simulink model "ES101A_DiagcMgr"  (R2013b)
settings: Solver=ode45  StartTime=0.0  StopTime=0.44  RelTol=1e-3
values from neighbouring files (symbols this model uses):
  BrdgVltg = DataDict.IpSignal    [ES101A_DiagcMgr_DataDict.m]
  DEM_CLEAR_PENDING = DataDict.Constant    [ES101A_DiagcMgr_DataDict.m]
  DEM_DTC_GROUP_ALL_DTCS = DataDict.Constant    [ES101A_DiagcMgr_DataDict.m]
  DFTAGICNTR_CNT_U08 = DataDict.Constant    [ES101A_DiagcMgr_DataDict.m]
  DIAGCMGR_NTCINFOSTSTESTFAILD_CNT_U08 = DataDict.Constant    [ES101A_DiagcMgrProxyX_DataDict.m]    (also in ES101A_DiagcMgr_DataDict.m)
  DIAGCMGR_NTCINFOSTSTESTFAILDTHISIGNCYC_CNT_U08 = DataDict.Constant    [ES101A_DiagcMgr_DataDict.m]
  DIAGCMGR_NTCINFOSTSTESTNOTCMPLTHISIGNCYC_CNT_U08 = DataDict.Constant    [ES101A_DiagcMgrProxyX_DataDict.m]    (also in ES101A_DiagcMgr_DataDict.m)
  DiagcMgrFltResp = DataDict.Calibration    [ES101A_DiagcMgrProxyX_DataDict.m]    (also in ES101A_DiagcMgr_DataDict.m)
  DiagcMgrNtcFltAry = DataDict.NVM    [ES101A_DiagcMgr_DataDict.m]
  DIAGCSTSCTRLDSHTDWNFLTPRSNT_CNT_U16 = DataDict.Constant    [ES101A_DiagcMgr_DataDict.m]
  DIAGCSTSDFTHWAG_CNT_U16 = DataDict.Constant    [ES101A_DiagcMgr_DataDict.m]
  DIAGCSTSDFTHWAGSERLCOMEXPRTVAL_CNT_U16 = DataDict.Constant    [ES101A_DiagcMgr_DataDict.m]
  DIAGCSTSDFTVEHSPD_CNT_U16 = DataDict.Constant    [ES101A_DiagcMgr_DataDict.m]
  DIAGCSTSININVAL_CNT_U16 = DataDict.Constant    [ES101A_DiagcMgrProxyX_DataDict.m]    (also in ES101A_DiagcMgr_DataDict.m)
  DIAGCSTSIVTR1INACTV_CNT_U16 = DataDict.Constant    [ES101A_DiagcMgr_DataDict.m]
  DIAGCSTSIVTR2INACTV_CNT_U16 = DataDict.Constant    [ES101A_DiagcMgr_DataDict.m]
  DIAGCSTSLIMDTPRFMNC_CNT_U16 = DataDict.Constant    [ES101A_DiagcMgr_DataDict.m]
  DIAGCSTSRAMPTOZEROFLTPRSNT_CNT_U16 = DataDict.Constant    [ES101A_DiagcMgr_DataDict.m]
  DIAGCSTSWHLIMBREJCTNDI_CNT_U16 = DataDict.Constant    [ES101A_DiagcMgr_DataDict.m]
  DTCIDXSTSFAIL_CNT_U08 = DataDict.Constant    [ES101A_DiagcMgr_DataDict.m]
  DTCIDXSTSNONTC_CNT_U08 = DataDict.Constant    [ES101A_DiagcMgr_DataDict.m]
  DTCIDXSTSNORES_CNT_U08 = DataDict.Constant    [ES101A_DiagcMgr_DataDict.m]
  DTCIDXSTSPASS_CNT_U08 = DataDict.Constant    [ES101A_DiagcMgr_DataDict.m]
  DTCIDXSTSUPDCFMD_CNT_U08 = DataDict.Constant    [ES101A_DiagcMgr_DataDict.m]
  ELECGLBPRM_IVTRCNT_CNT_U08 = DataDict.ConfigParam    [ES101A_DiagcMgrProxyX_DataDict.m]    (also in ES101A_DiagcMgr_DataDict.m)
  FLTINJ_DIAGCMGR_DIAGCSTSIVTR1INACTV = DataDict.Constant    [ES101A_DiagcMgr_DataDict.m]
  FLTINJ_DIAGCMGR_DIAGCSTSIVTR2INACTV = DataDict.Constant    [ES101A_DiagcMgr_DataDict.m]
  HwTq = DataDict.IpSignal    [ES101A_DiagcMgr_DataDict.m]
  IgnCntr = DataDict.IpSignal    [ES101A_DiagcMgr_DataDict.m]
  MAXDEBCNTRVAL_CNT_S16 = DataDict.Constant    [ES101A_DiagcMgr_DataDict.m]
  MAXRAMPRATE_ULSPERSEC_F32 = DataDict.Constant    [ES101A_DiagcMgrProxyX_DataDict.m]    (also in ES101A_DiagcMgr_DataDict.m)
  MINDEBCNTRVAL_CNT_S16 = DataDict.Constant    [ES101A_DiagcMgr_DataDict.m]
  MINRAMPRATE_ULSPERSEC_F32 = DataDict.Constant    [ES101A_DiagcMgrProxyX_DataDict.m]    (also in ES101A_DiagcMgr_DataDict.m)
  SCAMOTTQCMDTOONE_ULS_F32 = DataDict.Constant    [ES101A_DiagcMgrProxyX_DataDict.m]    (also in ES101A_DiagcMgr_DataDict.m)
  SCAMOTTQCMDTOZERO_ULS_F32 = DataDict.Constant    [ES101A_DiagcMgrProxyX_DataDict.m]    (also in ES101A_DiagcMgr_DataDict.m)
  SysSt = DataDict.IpSignal    [ES101A_DiagcMgr_DataDict.m]
  VehSpd = DataDict.IpSignal    [ES101A_DiagcMgr_DataDict.m]
undefined symbols (not defined in the file or in its folder): ActvMotTqCmdSca, ActvRampRate, AgiCntr, Dem_DTCFormatType, Dem_DTCOriginType, Dem_EventStatusType, DiagcData, DiagcMgrNtcMap, DiagcSts, DtcEnaMask, EcuT, HistNtcFltAry, MicroDiagcData, MotTq, NtcNr, NtcNrWithResd1, NtcStInfo, ProxySetNtcData, Sts, SysSt1, TOTNROFDTC_CNT_U08
libraries: simulink x149, FloatToFixd x5, NxtrNvM x3
(part 9 of 13)

== system ES101A_DiagcMgr/DiagcMgr/SetNtcStsCore/NtcNr is Valid/Diagnostics Not Inhibited/NtcEnabled/NTCSTS_PREPASSD/Update NtcInfoSts/Do Nothing ==
  Action Port : ActionPort  ActionType=else
  CopyRight2 : Subsystem  Description=|  mask(Copyright Information){none=on}
      | Copyright info block.                                               
      |                                                                     
      | Place copyright information at the top of every subsystem in design.
      mask prompts: none "No parameters"
      mask help: Place copyright information at the top of every subsystem in design.
      mask Display:
      | NxtrConf = 'Nexteer Confidential';
      | 
      | sys = bdroot; %handle for the current model ("system")
      | first = get_param(sys,'Created');
      | first = first(end-3:end);  %year is last four digits
      | 
      | last = get_param(sys,'LastModifiedDate');
      | if isempty(last)
      |     last = datestr(now,'yyyy');
      | else
      |     last = last(end-3:end);
      | end
      | 
      | if strcmp(first,last)
      |     fprintf('%s -- Copyright %s Nexteer',NxtrConf,first)
      | else
      |     fprintf('%s -- %s%s- %s Nexteer',NxtrConf,char(169),first,last)
      | end

== system ES101A_DiagcMgr/DiagcMgr/SetNtcStsCore/NtcNr is Valid/Diagnostics Not Inhibited/NtcEnabled/NTCSTS_PREPASSD/Update NtcInfoSts/Update NTC Info's Status Byte & Update the NTC Fault Array ==
  NtcInfo_ArgIn : Inport
  DebStep_ArgIn : Inport  Port=2
  NtcInfoDebCntr_ArgIn : Inport  Port=3
  Action Port : ActionPort  ActionType=then
  CopyRight2 : Subsystem  Description=|  mask(Copyright Information){none=on}
      | Copyright info block.                                               
      |                                                                     
      | Place copyright information at the top of every subsystem in design.
      mask prompts: none "No parameters"
      mask help: Place copyright information at the top of every subsystem in design.
      mask Display:
      | NxtrConf = 'Nexteer Confidential';
      | 
      | sys = bdroot; %handle for the current model ("system")
      | first = get_param(sys,'Created');
      | first = first(end-3:end);  %year is last four digits
      | 
      | last = get_param(sys,'LastModifiedDate');
      | if isempty(last)
      |     last = datestr(now,'yyyy');
      | else
      |     last = last(end-3:end);
      | end
      | 
      | if strcmp(first,last)
      |     fprintf('%s -- Copyright %s Nexteer',NxtrConf,first)
      | else
      |     fprintf('%s -- %s%s- %s Nexteer',NxtrConf,char(169),first,last)
      | end
  Decrement Counter : Subsystem  RequirementInfo="{'linktype_rmi_doors' '0000c474 (/ESG Group/FDD Module Requirements/EA4 Specific/ES101A_DiagcMgr)' '#ES101A_271' 'true' 'REQ:  ES101A_271' '' ; 'linktype_rmi_doors' '0000c474 (/ESG Group/FDD Module Requirements/EA4 Specific/ES101A_DiagcMgr)' '#ES101A_272' 'true' 'REQ:  ES101A_272' '' } %GIDa_7e8fb58f_d104_4b81_a44a_d0c429ffb579"  Priority=1  TreatAsAtomicUnit=on
      settings: AttributesFormatString=Priority = %<Priority>  RTWSystemCode=Inline
  "NtcInfo_ArgOut " : Outport
  NtcInfoDebCntr_ArgOut : Outport  Port=2
  wires:
  Decrement Counter/1(NtcInfo_ArgOut) -> "NtcInfo_ArgOut "/1
  DebStep_ArgIn/1 -> Decrement Counter/2(DebStep_ArgIn)
  NtcInfo_ArgIn/1 -> Decrement Counter/1("NtcInfo_ArgIn ")
  NtcInfoDebCntr_ArgIn/1 -> Decrement Counter/3(NtcInfoDebCntr_ArgIn)
  Decrement Counter/2(NtcInfoDebCntr_ArgOut) -> NtcInfoDebCntr_ArgOut/1

== system ES101A_DiagcMgr/DiagcMgr/DiagcMgrIninCore/Update NtcInfoAry From NvM/Update NtcInfoAry/Update NtcInfoAry Aging Counter And Confirmed Bit/If Action/Subsystem/0 < AgingCntr < 64/CopyRight2 ==

== system ES101A_DiagcMgr/DiagcMgr/DiagcMgrIninCore/Update NtcInfoAry From NvM/Update NtcInfoAry/Update NtcInfoAry Aging Counter And Confirmed Bit/If Action/Subsystem/AgingCntr >= 64 Do Nothing/CopyRight1 ==

== system ES101A_DiagcMgr/DiagcMgr/DiagcMgrPer2/Normal Periodic Processing/For All DTCs/For Each DTC/Check If DTC Status has Changed/DTC Status Changed OR DTC Update NOT Confirmed/Update DTC Index Previous Status with DTC Index Current Status/CopyRight2 ==

== system ES101A_DiagcMgr/DiagcMgr/DiagcMgrPer2/Normal Periodic Processing/For All DTCs/For Each DTC/Check If DTC Status has Changed/DTC Status Changed OR DTC Update NOT Confirmed/Update DTC Status/CopyRight2 ==

== system ES101A_DiagcMgr/DiagcMgr/DiagcMgrPer2/Normal Periodic Processing/For All DTCs/For Each DTC/Check If DTC Status has Changed/DTC Status Changed OR DTC Update NOT Confirmed/Update DTC Status/Dtc Status is Failed ==
  DtcIdx : Inport
  Action Port : ActionPort  ActionType=elseif
  Constant1 : Constant  Value=Dem_EventStatusType.DEM_EVENT_STATUS_FAILED
  CopyRight2 : Subsystem  Description=|  mask(Copyright Information){none=on}
      | Copyright info block.                                               
      |                                                                     
      | Place copyright information at the top of every subsystem in design.
      mask prompts: none "No parameters"
      mask help: Place copyright information at the top of every subsystem in design.
      mask Display:
      | NxtrConf = 'Nexteer Confidential';
      | 
      | sys = bdroot; %handle for the current model ("system")
      | first = get_param(sys,'Created');
      | first = first(end-3:end);  %year is last four digits
      | 
      | last = get_param(sys,'LastModifiedDate');
      | if isempty(last)
      |     last = datestr(now,'yyyy');
      | else
      |     last = last(end-3:end);
      | end
      | 
      | if strcmp(first,last)
      |     fprintf('%s -- Copyright %s Nexteer',NxtrConf,first)
      | else
      |     fprintf('%s -- %s%s- %s Nexteer',NxtrConf,char(169),first,last)
      | end
  Data Store Read : DataStoreRead  DataStoreName=DemDtcEveIdMap
  Dem_SetEventStatus : Subsystem
  Selector2 : Selector  IndexMode=Zero-based  InputPortWidth=14  IndexOptions=Index vector (port)  Indices=[1 3]  OutputSizes=1
  Update 'DTC Index Update Confirmed' Bit : Subsystem
  wires:
  Dem_SetEventStatus/1(Dem_SetEventStatus_StdRtn) -> Update 'DTC Index Update Confirmed' Bit/1(Dem_SetEventStatus_StdRtn)
  Constant1/1 -> Dem_SetEventStatus/2(EventStatus), Update 'DTC Index Update Confirmed' Bit/2(DtcIdxPrevSts)
  Data Store Read/1 -> Selector2/1
  Selector2/1 -> Dem_SetEventStatus/1(EventId)
  DtcIdx/1 -> Selector2/2, Update 'DTC Index Update Confirmed' Bit/3(DtcIdx)

== system ES101A_DiagcMgr/DiagcMgr/DiagcMgrPer2/Normal Periodic Processing/For All DTCs/For Each DTC/Check If DTC Status has Changed/DTC Status Changed OR DTC Update NOT Confirmed/Update DTC Status/Dtc Status is No Result or No Ntc ==
  DtcIdx : Inport
  Action Port : ActionPort
  Assignment : Assignment  IndexMode=Zero-based  IndexOptions=Starting index (port)  Indices=1  OutputSizes=1
  CopyRight2 : Subsystem  Description=|  mask(Copyright Information){none=on}
      | Copyright info block.                                               
      |                                                                     
      | Place copyright information at the top of every subsystem in design.
      mask prompts: none "No parameters"
      mask help: Place copyright information at the top of every subsystem in design.
      mask Display:
      | NxtrConf = 'Nexteer Confidential';
      | 
      | sys = bdroot; %handle for the current model ("system")
      | first = get_param(sys,'Created');
      | first = first(end-3:end);  %year is last four digits
      | 
      | last = get_param(sys,'LastModifiedDate');
      | if isempty(last)
      |     last = datestr(now,'yyyy');
      | else
      |     last = last(end-3:end);
      | end
      | 
      | if strcmp(first,last)
      |     fprintf('%s -- Copyright %s Nexteer',NxtrConf,first)
      | else
      |     fprintf('%s -- %s%s- %s Nexteer',NxtrConf,char(169),first,last)
      | end
  Data Store Read : DataStoreRead  DataStoreName=DtcIdxPrevSts
  Data Store Read1 : DataStoreRead  DataStoreName=DtcIdxPrevSts
  Data Store Write : DataStoreWrite  DataStoreName=DtcIdxPrevSts
  Set Bit 7 (DTC Update Confirmed) : Subsystem
  wires:
  Data Store Read/1 -> Assignment/1
  Assignment/1 -> Data Store Write/1
  DtcIdx/1 -> Assignment/3
  Data Store Read1/1 -> Set Bit 7 (DTC Update Confirmed)/1(In1)
  Set Bit 7 (DTC Update Confirmed)/1(Out1) -> Assignment/2

== system ES101A_DiagcMgr/DiagcMgr/DiagcMgrPer2/Normal Periodic Processing/For All DTCs/For Each DTC/Check If DTC Status has Changed/DTC Status Changed OR DTC Update NOT Confirmed/Update DTC Status/Dtc Status is Passed ==
  DtcIdx : Inport
  Action Port : ActionPort
  Constant : Constant  Value=Dem_EventStatusType.DEM_EVENT_STATUS_PASSED
  CopyRight2 : Subsystem  Description=|  mask(Copyright Information){none=on}
      | Copyright info block.                                               
      |                                                                     
      | Place copyright information at the top of every subsystem in design.
      mask prompts: none "No parameters"
      mask help: Place copyright information at the top of every subsystem in design.
      mask Display:
      | NxtrConf = 'Nexteer Confidential';
      | 
      | sys = bdroot; %handle for the current model ("system")
      | first = get_param(sys,'Created');
      | first = first(end-3:end);  %year is last four digits
      | 
      | last = get_param(sys,'LastModifiedDate');
      | if isempty(last)
      |     last = datestr(now,'yyyy');
      | else
      |     last = last(end-3:end);
      | end
      | 
      | if strcmp(first,last)
      |     fprintf('%s -- Copyright %s Nexteer',NxtrConf,first)
      | else
      |     fprintf('%s -- %s%s- %s Nexteer',NxtrConf,char(169),first,last)
      | end
  Data Store Read : DataStoreRead  DataStoreName=DemDtcEveIdMap
  Dem_SetEventStatus : Subsystem
  Selector2 : Selector  IndexMode=Zero-based  InputPortWidth=14  IndexOptions=Index vector (port)  Indices=[1 3]  OutputSizes=1
  Update 'DTC Index Update Confirmed' Bit : Subsystem
  wires:
  Constant/1 -> Update 'DTC Index Update Confirmed' Bit/2(DtcIdxPrevSts), Dem_SetEventStatus/2(EventStatus)
  Dem_SetEventStatus/1(Dem_SetEventStatus_StdRtn) -> Update 'DTC Index Update Confirmed' Bit/1(Dem_SetEventStatus_StdRtn)
  DtcIdx/1 -> Update 'DTC Index Update Confirmed' Bit/3(DtcIdx), Selector2/2
  Selector2/1 -> Dem_SetEventStatus/1(EventId)
  Data Store Read/1 -> Selector2/1

== system ES101A_DiagcMgr/DiagcMgr/DiagcMgrPer2/Normal Periodic Processing/For All NTCs/For Each NTC/Update DTC Status/NTC Enabled/DTC Fail/CopyRight2 ==

== system ES101A_DiagcMgr/DiagcMgr/DiagcMgrPer2/Normal Periodic Processing/For All NTCs/For Each NTC/Update DTC Status/NTC Enabled/DTC NoRes/CopyRight2 ==

== system ES101A_DiagcMgr/DiagcMgr/DiagcMgrPer2/Normal Periodic Processing/For All NTCs/For Each NTC/Update DTC Status/NTC Enabled/DTC Pass/CopyRight2 ==

== system ES101A_DiagcMgr/DiagcMgr/DiagcMgrPer2/Normal Periodic Processing/For All NTCs/For Each NTC/Update DTC Status/NTC Enabled/Do Nothing/CopyRight2 ==

== system ES101A_DiagcMgr/DiagcMgr/SetNtcStsCore/NtcNr is Valid/Diagnostics Not Inhibited/NtcEnabled/NTCSTS_FAILD/Update ISO Bits, Parameter Byte and AgiCntr /ProcessRampResponse and DiagcSts/ControlledShutdown Fault ==
  DiagcData_ArgIn : Inport
  ProxySetNtcData_ArgIn : Inport  Port=2
  TmpDiagcSts : Inport  Port=3
  Action Port : ActionPort
  Atomic Section2 : Subsystem  Description=|  RequirementInfo="{'linktype_rmi_doors' '0000c474 (/ESG Group/FDD Module Requirements/EA4 Specific/ES101A_DiagcMgr)' '#ES101A_300' 'true' 'REQ:  ES101A_300' '' } %GIDa_2bc6450b_700c_4982_9445_5c86aef287c5"
      | EXCLUSIVE AREA:
      | Write data into the DiagcSts Register & ActvRampRate Register
      settings: AttributesFormatString=%<Description>
  Bitwise Operator : simulink/Logic and Bit Operations/Bitwise Operator  logicop=OR  UseBitMask=off  NumInputPorts=3  BitMask=bin2dec('11011001')  BitMaskRealWorld=Stored Integer
  CopyRight2 : Subsystem  Description=|  mask(Copyright Information){none=on}
      | Copyright info block.                                               
      |                                                                     
      | Place copyright information at the top of every subsystem in design.
      mask prompts: none "No parameters"
      mask help: Place copyright information at the top of every subsystem in design.
      mask Display:
      | NxtrConf = 'Nexteer Confidential';
      | 
      | sys = bdroot; %handle for the current model ("system")
      | first = get_param(sys,'Created');
      | first = first(end-3:end);  %year is last four digits
      | 
      | last = get_param(sys,'LastModifiedDate');
      | if isempty(last)
      |     last = datestr(now,'yyyy');
      | else
      |     last = last(end-3:end);
      | end
      | 
      | if strcmp(first,last)
      |     fprintf('%s -- Copyright %s Nexteer',NxtrConf,first)
      | else
      |     fprintf('%s -- %s%s- %s Nexteer',NxtrConf,char(169),first,last)
      | end
  Diagnostic Status Controlled Shutdown Fault Present : Constant  Value=DIAGCSTSCTRLDSHTDWNFLTPRSNT_CNT_U16
  Ramp To Zero Fault Present : Constant  Value=DIAGCSTSRAMPTOZEROFLTPRSNT_CNT_U16  OutDataTypeStr=uint16
  DiagcData_ArgOut : Outport
  ProxySetNtcData_ArgOut : Outport  Port=2
  wires:
  Diagnostic Status Controlled Shutdown Fault Present/1 -> Bitwise Operator/1
  Ramp To Zero Fault Present/1 -> Bitwise Operator/2
  Bitwise Operator/1 -> Atomic Section2/1(TmpDiagcSts)
  DiagcData_ArgIn/1 -> Atomic Section2/2(DiagcData_ArgInOut)
  ProxySetNtcData_ArgIn/1 -> Atomic Section2/3(ProxySetNtcData_ArgInOut)
  Atomic Section2/1(DiagcData_ArgOut) -> DiagcData_ArgOut/1
  Atomic Section2/2(ProxySetNtcData_ArgOut) -> ProxySetNtcData_ArgOut/1
  TmpDiagcSts/1 -> Bitwise Operator/3

== system ES101A_DiagcMgr/DiagcMgr/SetNtcStsCore/NtcNr is Valid/Diagnostics Not Inhibited/NtcEnabled/NTCSTS_FAILD/Update ISO Bits, Parameter Byte and AgiCntr /ProcessRampResponse and DiagcSts/CopyRight2 ==

== system ES101A_DiagcMgr/DiagcMgr/SetNtcStsCore/NtcNr is Valid/Diagnostics Not Inhibited/NtcEnabled/NTCSTS_FAILD/Update ISO Bits, Parameter Byte and AgiCntr /ProcessRampResponse and DiagcSts/InformationOnly Fault ==
  DiagcData_ArgIn : Inport
  ProxySetNtcData_ArgIn : Inport  Port=2
  TmpDiagcSts : Inport  Port=3
  Action Port : ActionPort
  Atomic Section2 : Subsystem  Description=|  RequirementInfo="{'linktype_rmi_doors' '0000c474 (/ESG Group/FDD Module Requirements/EA4 Specific/ES101A_DiagcMgr)' '#ES101A_300' 'true' 'REQ:  ES101A_300' '' } %GIDa_9448650f_4c83_4875_bae7_9fccd1156efd"
      | EXCLUSIVE AREA:
      | Write data into the DiagcSts Register & ActvRampRate Register
      settings: AttributesFormatString=%<Description>
  CopyRight2 : Subsystem  Description=|  mask(Copyright Information){none=on}
      | Copyright info block.                                               
      |                                                                     
      | Place copyright information at the top of every subsystem in design.
      mask prompts: none "No parameters"
      mask help: Place copyright information at the top of every subsystem in design.
      mask Display:
      | NxtrConf = 'Nexteer Confidential';
      | 
      | sys = bdroot; %handle for the current model ("system")
      | first = get_param(sys,'Created');
      | first = first(end-3:end);  %year is last four digits
      | 
      | last = get_param(sys,'LastModifiedDate');
      | if isempty(last)
      |     last = datestr(now,'yyyy');
      | else
      |     last = last(end-3:end);
      | end
      | 
      | if strcmp(first,last)
      |     fprintf('%s -- Copyright %s Nexteer',NxtrConf,first)
      | else
      |     fprintf('%s -- %s%s- %s Nexteer',NxtrConf,char(169),first,last)
      | end
  DiagcData_ArgOut : Outport
  ProxySetNtcData_ArgOut : Outport  Port=2
  wires:
  DiagcData_ArgIn/1 -> Atomic Section2/1(DiagcData_ArgInOut)
  ProxySetNtcData_ArgIn/1 -> Atomic Section2/2(ProxySetNtcData_ArgInOut)
  Atomic Section2/1(DiagcData_ArgOut) -> DiagcData_ArgOut/1
  Atomic Section2/2(ProxySetNtcData_ArgOut) -> ProxySetNtcData_ArgOut/1
  TmpDiagcSts/1 -> Atomic Section2/3(TmpDiagcSts)

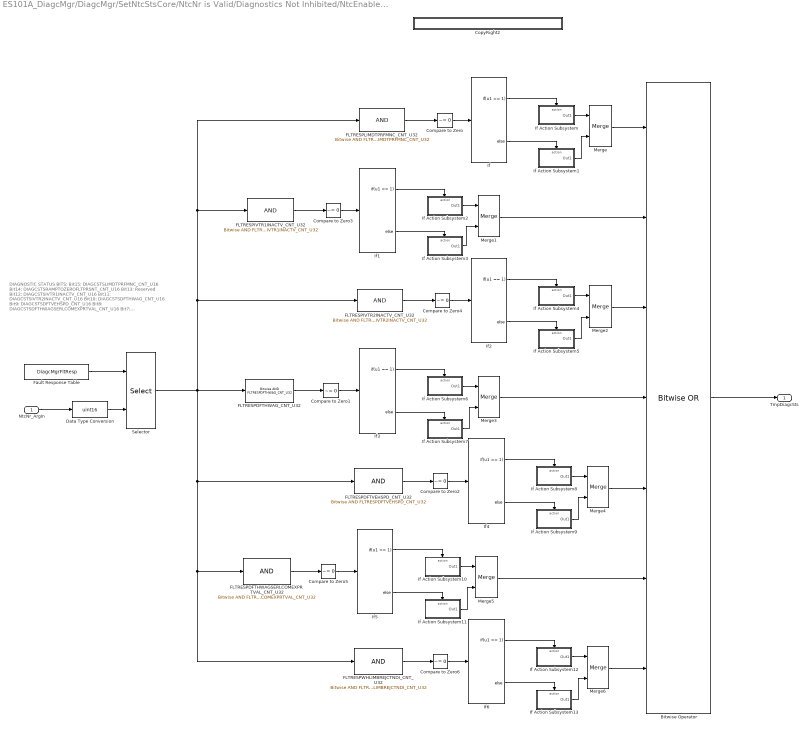
== system ES101A_DiagcMgr/DiagcMgr/SetNtcStsCore/NtcNr is Valid/Diagnostics Not Inhibited/NtcEnabled/NTCSTS_FAILD/Update ISO Bits, Parameter Byte and AgiCntr /ProcessRampResponse and DiagcSts/ProcessDiagcSts ==
  note: DIAGNOSTIC  STATUS  BITS:
      |
      | Bit15: DIAGCSTSLIMDTPRFMNC_CNT_U16
      | Bit14: DIAGCSTSRAMPTOZEROFLTPRSNT_CNT_U16
      | Bit13: Reserved
      | Bit12: DIAGCSTSIVTR1INACTV_CNT_U16
      | Bit11: DIAGCSTSIVTR2INACTV_CNT_U16
      | Bit10: DIAGCSTSDFTHWAG_CNT_U16
      | Bit9:   DIAGCSTSDFTVEHSPD_CNT_U16
      | Bit8:   DIAGCSTSDFTHWAGSERLCOMEXPRTVAL_CNT_U16
      | Bit7:   DIAGCSTSWHLIMBREJCTNDI_CNT_U16
      | Bit6:	   DIAGCSTSCTRLDIRAMP_CNT_U16
  NtcNr_ArgIn : Inport
  Bitwise Operator : simulink/Logic and Bit Operations/Bitwise Operator  logicop=OR  UseBitMask=off  NumInputPorts=7  BitMask=bin2dec('11011001')  BitMaskRealWorld=Stored Integer
  Compare to Zero{,1..6} (7 alike) : simulink/Logic and Bit Operations/Compare To Zero  relop=~=  OutDataTypeStr=boolean
  CopyRight2 : Subsystem  Description=|  mask(Copyright Information){none=on}
      | Copyright info block.                                               
      |                                                                     
      | Place copyright information at the top of every subsystem in design.
      mask prompts: none "No parameters"
      mask help: Place copyright information at the top of every subsystem in design.
      mask Display:
      | NxtrConf = 'Nexteer Confidential';
      | 
      | sys = bdroot; %handle for the current model ("system")
      | first = get_param(sys,'Created');
      | first = first(end-3:end);  %year is last four digits
      | 
      | last = get_param(sys,'LastModifiedDate');
      | if isempty(last)
      |     last = datestr(now,'yyyy');
      | else
      |     last = last(end-3:end);
      | end
      | 
      | if strcmp(first,last)
      |     fprintf('%s -- Copyright %s Nexteer',NxtrConf,first)
      | else
      |     fprintf('%s -- %s%s- %s Nexteer',NxtrConf,char(169),first,last)
      | end
  Data Type Conversion : DataTypeConversion  OutDataTypeStr=uint16
  FLTRESPDFTHWAGSERLCOMEXPRTVAL_CNT_U32 : simulink/Logic and Bit Operations/Bitwise Operator  logicop=AND  UseBitMask=on  BitMask=FLTRESPDFTHWAGSERLCOMEXPRTVAL_CNT_U32  BitMaskRealWorld=Stored Integer
  FLTRESPDFTHWAG_CNT_U32 : simulink/Logic and Bit Operations/Bitwise Operator  logicop=AND  UseBitMask=on  BitMask=FLTRESPDFTHWAG_CNT_U32  BitMaskRealWorld=Stored Integer
  FLTRESPDFTVEHSPD_CNT_U32 : simulink/Logic and Bit Operations/Bitwise Operator  logicop=AND  UseBitMask=on  BitMask=FLTRESPDFTVEHSPD_CNT_U32  BitMaskRealWorld=Stored Integer
  FLTRESPIVTR1INACTV_CNT_U32 : simulink/Logic and Bit Operations/Bitwise Operator  RequirementInfo={} %GIDa_da088e71_cf55_4258_9e23_348948e7cf64  logicop=AND  UseBitMask=on  BitMask=FLTRESPIVTR1INACTV_CNT_U32  BitMaskRealWorld=Stored Integer
  FLTRESPIVTR2INACTV_CNT_U32 : simulink/Logic and Bit Operations/Bitwise Operator  RequirementInfo={} %GIDa_49040b40_7700_4617_a7b3_5f9f919de844  logicop=AND  UseBitMask=on  BitMask=FLTRESPIVTR2INACTV_CNT_U32  BitMaskRealWorld=Stored Integer
  FLTRESPLIMDTPRFMNC_CNT_U32 : simulink/Logic and Bit Operations/Bitwise Operator  RequirementInfo={} %GIDa_3a19e481_3aa4_478f_99c0_cab30f84ef14  logicop=AND  UseBitMask=on  BitMask=FLTRESPLIMDTPRFMNC_CNT_U32  BitMaskRealWorld=Stored Integer
  FLTRESPWHLIMBREJCTNDI_CNT_U32 : simulink/Logic and Bit Operations/Bitwise Operator  logicop=AND  UseBitMask=on  BitMask=FLTRESPWHLIMBREJCTNDI_CNT_U32  BitMaskRealWorld=Stored Integer
  Fault Response Table : Constant  Value=DiagcMgrFltResp
  If{,1..6} (7 alike) : If  IfExpression=u1 == 1
  If Action Subsystem : Subsystem  TreatAsAtomicUnit=on
  If Action Subsystem1 : Subsystem  TreatAsAtomicUnit=on
  If Action Subsystem10 : Subsystem  TreatAsAtomicUnit=on
  If Action Subsystem11 : Subsystem  TreatAsAtomicUnit=on
  If Action Subsystem12 : Subsystem  TreatAsAtomicUnit=on
  If Action Subsystem13 : Subsystem  TreatAsAtomicUnit=on
  If Action Subsystem2 : Subsystem  TreatAsAtomicUnit=on
  If Action Subsystem3 : Subsystem  TreatAsAtomicUnit=on
  If Action Subsystem4 : Subsystem  TreatAsAtomicUnit=on
  If Action Subsystem5 : Subsystem  TreatAsAtomicUnit=on
  If Action Subsystem6 : Subsystem  TreatAsAtomicUnit=on
  If Action Subsystem7 : Subsystem  TreatAsAtomicUnit=on
  If Action Subsystem8 : Subsystem  TreatAsAtomicUnit=on
  If Action Subsystem9 : Subsystem  TreatAsAtomicUnit=on
  Merge{,1..6} (7 alike) : Merge
  Selector : Selector  IndexMode=Zero-based  InputPortWidth=512  IndexOptions=Index vector (port)  Indices=[1 3]  OutputSizes=1
  TmpDiagcSts : Outport
  wires:
  Compare to Zero4/1 -> If2/1
  Merge2/1 -> Bitwise Operator/3
  If Action Subsystem5/1(Out1) -> Merge2/2
  If Action Subsystem4/1(Out1) -> Merge2/1
  If2/2 -> If Action Subsystem5/Action
  If2/1 -> If Action Subsystem4/Action
  Merge1/1 -> Bitwise Operator/2
  Compare to Zero3/1 -> If1/1
  If Action Subsystem3/1(Out1) -> Merge1/2
  If Action Subsystem2/1(Out1) -> Merge1/1
  If1/2 -> If Action Subsystem3/Action
  If1/1 -> If Action Subsystem2/Action
  Merge/1 -> Bitwise Operator/1
  If Action Subsystem1/1(Out1) -> Merge/2
  If Action Subsystem/1(Out1) -> Merge/1
  Compare to Zero/1 -> If/1
  If/2 -> If Action Subsystem1/Action
  If/1 -> If Action Subsystem/Action
  Bitwise Operator/1 -> TmpDiagcSts/1
  FLTRESPIVTR2INACTV_CNT_U32/1 -> Compare to Zero4/1
  FLTRESPIVTR1INACTV_CNT_U32/1 -> Compare to Zero3/1
  Selector/1 -> FLTRESPWHLIMBREJCTNDI_CNT_U32/1, FLTRESPDFTHWAGSERLCOMEXPRTVAL_CNT_U32/1, FLTRESPDFTVEHSPD_CNT_U32/1, FLTRESPDFTHWAG_CNT_U32/1, FLTRESPLIMDTPRFMNC_CNT_U32/1, FLTRESPIVTR1INACTV_CNT_U32/1, FLTRESPIVTR2INACTV_CNT_U32/1
  Fault Response Table/1 -> Selector/1
  NtcNr_ArgIn/1 -> Data Type Conversion/1
  FLTRESPLIMDTPRFMNC_CNT_U32/1 -> Compare to Zero/1
  Compare to Zero1/1 -> If3/1
  Merge3/1 -> Bitwise Operator/4
  If Action Subsystem7/1(Out1) -> Merge3/2
  If Action Subsystem6/1(Out1) -> Merge3/1
  If3/2 -> If Action Subsystem7/Action
  If3/1 -> If Action Subsystem6/Action
  FLTRESPDFTHWAG_CNT_U32/1 -> Compare to Zero1/1
  Compare to Zero2/1 -> If4/1
  Merge4/1 -> Bitwise Operator/5
  If Action Subsystem9/1(Out1) -> Merge4/2
  If Action Subsystem8/1(Out1) -> Merge4/1
  If4/2 -> If Action Subsystem9/Action
  If4/1 -> If Action Subsystem8/Action
  FLTRESPDFTVEHSPD_CNT_U32/1 -> Compare to Zero2/1
  Compare to Zero5/1 -> If5/1
  Merge5/1 -> Bitwise Operator/6
  If Action Subsystem11/1(Out1) -> Merge5/2
  If Action Subsystem10/1(Out1) -> Merge5/1
  If5/2 -> If Action Subsystem11/Action
  If5/1 -> If Action Subsystem10/Action
  FLTRESPDFTHWAGSERLCOMEXPRTVAL_CNT_U32/1 -> Compare to Zero5/1
  Compare to Zero6/1 -> If6/1
  Merge6/1 -> Bitwise Operator/7
  If Action Subsystem13/1(Out1) -> Merge6/2
  If Action Subsystem12/1(Out1) -> Merge6/1
  If6/2 -> If Action Subsystem13/Action
  If6/1 -> If Action Subsystem12/Action
  FLTRESPWHLIMBREJCTNDI_CNT_U32/1 -> Compare to Zero6/1
  Data Type Conversion/1 -> Selector/2

== system ES101A_DiagcMgr/DiagcMgr/SetNtcStsCore/NtcNr is Valid/Diagnostics Not Inhibited/NtcEnabled/NTCSTS_FAILD/Update ISO Bits, Parameter Byte and AgiCntr /ProcessRampResponse and DiagcSts/RapidShutdown Fault ==
  DiagcData_ArgIn : Inport
  ProxySetNtcData_ArgIn : Inport  Port=2
  TmpDiagcSts : Inport  Port=3
  Action Port : ActionPort
  Atomic Section2 : Subsystem  Description=|  RequirementInfo="{'linktype_rmi_doors' '0000c474 (/ESG Group/FDD Module Requirements/EA4 Specific/ES101A_DiagcMgr)' '#ES101A_300' 'true' 'REQ:  ES101A_300' '' } %GIDa_00cb0b6f_e255_4c4e_bed6_f3cda34ac4d2"
      | EXCLUSIVE AREA:
      | Write data into the DiagcSts Register & ActvRampRate Register
      settings: AttributesFormatString=%<Description>
  Bitwise Operator : simulink/Logic and Bit Operations/Bitwise Operator  logicop=OR  UseBitMask=off  NumInputPorts=2  BitMask=bin2dec('11011001')  BitMaskRealWorld=Stored Integer
  CopyRight2 : Subsystem  Description=|  mask(Copyright Information){none=on}
      | Copyright info block.                                               
      |                                                                     
      | Place copyright information at the top of every subsystem in design.
      mask prompts: none "No parameters"
      mask help: Place copyright information at the top of every subsystem in design.
      mask Display:
      | NxtrConf = 'Nexteer Confidential';
      | 
      | sys = bdroot; %handle for the current model ("system")
      | first = get_param(sys,'Created');
      | first = first(end-3:end);  %year is last four digits
      | 
      | last = get_param(sys,'LastModifiedDate');
      | if isempty(last)
      |     last = datestr(now,'yyyy');
      | else
      |     last = last(end-3:end);
      | end
      | 
      | if strcmp(first,last)
      |     fprintf('%s -- Copyright %s Nexteer',NxtrConf,first)
      | else
      |     fprintf('%s -- %s%s- %s Nexteer',NxtrConf,char(169),first,last)
      | end
  Ramp To Zero Fault Present1 : Constant  Value=DIAGCSTSRAMPTOZEROFLTPRSNT_CNT_U16  OutDataTypeStr=uint16
  "DiagcData_ArgOut " : Outport
  "ProxySetNtcData_ArgOut " : Outport  Port=2
  wires:
  Ramp To Zero Fault Present1/1 -> Bitwise Operator/1
  Bitwise Operator/1 -> Atomic Section2/1(TmpDiagcSts)
  TmpDiagcSts/1 -> Bitwise Operator/2
  DiagcData_ArgIn/1 -> Atomic Section2/2(DiagcData_ArgIn)
  ProxySetNtcData_ArgIn/1 -> Atomic Section2/3(ProxySetNtcData_ArgIn)
  Atomic Section2/1("DiagcData_ArgInOut ") -> "DiagcData_ArgOut "/1
  Atomic Section2/2("ProxySetNtcData_ArgOut ") -> "ProxySetNtcData_ArgOut "/1

== system ES101A_DiagcMgr/DiagcMgr/SetNtcStsCore/NtcNr is Valid/Diagnostics Not Inhibited/NtcEnabled/NTCSTS_FAILD/Update ISO Bits, Parameter Byte and AgiCntr /ProcessRampResponse and DiagcSts/TimedShutdown Fault ==
  FaultResponseRampBits : Inport
  DiagcData_ArgIn : Inport  Port=2
  ProxySetNtcData_ArgIn : Inport  Port=3
  TmpDiagcSts : Inport  Port=4
  Action Port : ActionPort
  Atomic Section2 : Subsystem  Description=|  RequirementInfo="{'linktype_rmi_doors' '0000c474 (/ESG Group/FDD Module Requirements/EA4 Specific/ES101A_DiagcMgr)' '#ES101A_300' 'true' 'REQ:  ES101A_300' '' } %GIDa_f2b36a2b_7d5b_48dc_b948_a7ca95944c5c"
      | EXCLUSIVE AREA:
      | Write data into the DiagcSts Register & ActvRampRate Register
      settings: AttributesFormatString=%<Description>
  Bitwise Operator : simulink/Logic and Bit Operations/Bitwise Operator  logicop=OR  UseBitMask=off  NumInputPorts=2  BitMask=bin2dec('11011001')  BitMaskRealWorld=Stored Integer
  CopyRight2 : Subsystem  Description=|  mask(Copyright Information){none=on}
      | Copyright info block.                                               
      |                                                                     
      | Place copyright information at the top of every subsystem in design.
      mask prompts: none "No parameters"
      mask help: Place copyright information at the top of every subsystem in design.
      mask Display:
      | NxtrConf = 'Nexteer Confidential';
      | 
      | sys = bdroot; %handle for the current model ("system")
      | first = get_param(sys,'Created');
      | first = first(end-3:end);  %year is last four digits
      | 
      | last = get_param(sys,'LastModifiedDate');
      | if isempty(last)
      |     last = datestr(now,'yyyy');
      | else
      |     last = last(end-3:end);
      | end
      | 
      | if strcmp(first,last)
      |     fprintf('%s -- Copyright %s Nexteer',NxtrConf,first)
      | else
      |     fprintf('%s -- %s%s- %s Nexteer',NxtrConf,char(169),first,last)
      | end
  Direct Lookup Table (n-D)1 : LookupNDDirect  NumberOfTableDimensions=1  Table=[0.1,0.125,0.1428,0.1667,0.2,0.25,0.333,0.5,1,2,3.333,10,500]  TableDataTypeStr=single
  Ramp To Zero Fault Present : Constant  Value=DIAGCSTSRAMPTOZEROFLTPRSNT_CNT_U16  OutDataTypeStr=uint16
  DiagcData_ArgOut : Outport
  ProxySetNtcData_ArgOut : Outport  Port=2
  wires:
  Ramp To Zero Fault Present/1 -> Bitwise Operator/1
  FaultResponseRampBits/1 -> Direct Lookup Table (n-D)1/1
  Direct Lookup Table (n-D)1/1 -> Atomic Section2/2(RampRate)
  Atomic Section2/1(DiagcData_ArgOut) -> DiagcData_ArgOut/1
  Atomic Section2/2(ProxySetNtcData_ArgOut) -> ProxySetNtcData_ArgOut/1
  DiagcData_ArgIn/1 -> Atomic Section2/3(DiagcData_ArgIn)
  ProxySetNtcData_ArgIn/1 -> Atomic Section2/4(ProxySetNtcData_ArgIn)
  Bitwise Operator/1 -> Atomic Section2/1(TmpDiagcSts)
  TmpDiagcSts/1 -> Bitwise Operator/2

== system ES101A_DiagcMgr/DiagcMgr/SetNtcStsCore/NtcNr is Valid/Diagnostics Not Inhibited/NtcEnabled/NTCSTS_FAILD/Update ISO Bits, Parameter Byte and AgiCntr /UpdSnpshtData/CopyRight1 ==

== system ES101A_DiagcMgr/DiagcMgr/SetNtcStsCore/NtcNr is Valid/Diagnostics Not Inhibited/NtcEnabled/NTCSTS_FAILD/Update ISO Bits, Parameter Byte and AgiCntr /UpdSnpshtData/Snapshot Data Enabled ==
  NtcNr : Inport
  NtcStInfo : Inport  Port=2
  SnapshotDataBus : Inport  Port=3
  Action Port : ActionPort  ActionType=then
  CopyRight2 : Subsystem  Description=|  mask(Copyright Information){none=on}
      | Copyright info block.                                               
      |                                                                     
      | Place copyright information at the top of every subsystem in design.
      mask prompts: none "No parameters"
      mask help: Place copyright information at the top of every subsystem in design.
      mask Display:
      | NxtrConf = 'Nexteer Confidential';
      | 
      | sys = bdroot; %handle for the current model ("system")
      | first = get_param(sys,'Created');
      | first = first(end-3:end);  %year is last four digits
      | 
      | last = get_param(sys,'LastModifiedDate');
      | if isempty(last)
      |     last = datestr(now,'yyyy');
      | else
      |     last = last(end-3:end);
      | end
      | 
      | if strcmp(first,last)
      |     fprintf('%s -- Copyright %s Nexteer',NxtrConf,first)
      | else
      |     fprintf('%s -- %s%s- %s Nexteer',NxtrConf,char(169),first,last)
      | end
  Initialize : Subsystem  Priority=1
      settings: AttributesFormatString=Priority = %<Priority>
  Temp: Snapshot Data Array Index : DataStoreMemory  RequirementInfo={} %GIDa_fea31163_adab_4e6e_b96c_8919633de4bc  DataStoreName=SnpshtDataAryIdx  OutDataTypeStr=uint8  Dimensions=20
  Temp: Snapshot Data Array Index Invalid : DataStoreMemory  RequirementInfo={} %GIDa_e5173b47_1007_42ec_a928_99d407331b98  DataStoreName=SnpshtDataAryIdxInvld  InitialValue=1  OutDataTypeStr=boolean  Dimensions=20
  "While " : Subsystem  Priority=2
      settings: AttributesFormatString=Priority = %<Priority>
  wires:
  NtcNr/1 -> "While "/1(NtcNr)
  NtcStInfo/1 -> "While "/2(NtcStInfo)
  SnapshotDataBus/1 -> "While "/3(SnapshotDataBus)

== system ES101A_DiagcMgr/DiagcMgr/SetNtcStsCore/NtcNr is Valid/Diagnostics Not Inhibited/NtcEnabled/NTCSTS_FAILD/Update ISO Bits, Parameter Byte and AgiCntr /Update ISO Bits, Parameter Byte and AgiCntr/Clear: DIAGCMGR_NTCINFOSTSTESTNOTCMPLTHISIGNCYC_CNT_U08 ==
  In2 : Inport
  In1 : Inport  Port=2
  Bitwise Operator : simulink/Logic and Bit Operations/Bitwise Operator  logicop=NOT  UseBitMask=off  BitMask=bin2dec('11011001')  BitMaskRealWorld=Stored Integer
  Bitwise Operator1 : simulink/Logic and Bit Operations/Bitwise Operator  logicop=AND  UseBitMask=off  NumInputPorts=2  BitMask=bin2dec('11011001')  BitMaskRealWorld=Stored Integer
  Out1 : Outport
  wires:
  Bitwise Operator1/1 -> Out1/1
  In2/1 -> Bitwise Operator1/1
  In1/1 -> Bitwise Operator/1
  Bitwise Operator/1 -> Bitwise Operator1/2

== system ES101A_DiagcMgr/DiagcMgr/SetNtcStsCore/NtcNr is Valid/Diagnostics Not Inhibited/NtcEnabled/NTCSTS_FAILD/Update ISO Bits, Parameter Byte and AgiCntr /Update ISO Bits, Parameter Byte and AgiCntr/CopyRight2 ==

== system ES101A_DiagcMgr/DiagcMgr/SetNtcStsCore/NtcNr is Valid/Diagnostics Not Inhibited/NtcEnabled/NTCSTS_PASSD/Update NtcInfoSts /Do Nothing/CopyRight2 ==

== system ES101A_DiagcMgr/DiagcMgr/SetNtcStsCore/NtcNr is Valid/Diagnostics Not Inhibited/NtcEnabled/NTCSTS_PASSD/Update NtcInfoSts /Update NTC Info's Status Byte/Clear: DIAGCMGR_NTCINFOSTSTESTFAILD_CNT_U08 ==
  In2 : Inport
  In1 : Inport  Port=2
  Bitwise Operator : simulink/Logic and Bit Operations/Bitwise Operator  logicop=NOT  UseBitMask=off  BitMask=bin2dec('11011001')  BitMaskRealWorld=Stored Integer
  Bitwise Operator1 : simulink/Logic and Bit Operations/Bitwise Operator  logicop=AND  UseBitMask=off  NumInputPorts=2  BitMask=bin2dec('11011001')  BitMaskRealWorld=Stored Integer
  Out1 : Outport
  wires:
  Bitwise Operator/1 -> Bitwise Operator1/2
  In1/1 -> Bitwise Operator/1
  In2/1 -> Bitwise Operator1/1
  Bitwise Operator1/1 -> Out1/1

== system ES101A_DiagcMgr/DiagcMgr/SetNtcStsCore/NtcNr is Valid/Diagnostics Not Inhibited/NtcEnabled/NTCSTS_PASSD/Update NtcInfoSts /Update NTC Info's Status Byte/Clear: DIAGCMGR_NTCINFOSTSTESTNOTCMPLTHISIGNCYC_CNT_U08 ==
  In2 : Inport
  In1 : Inport  Port=2
  Bitwise Operator : simulink/Logic and Bit Operations/Bitwise Operator  logicop=NOT  UseBitMask=off  BitMask=bin2dec('11011001')  BitMaskRealWorld=Stored Integer
  Bitwise Operator1 : simulink/Logic and Bit Operations/Bitwise Operator  logicop=AND  UseBitMask=off  NumInputPorts=2  BitMask=bin2dec('11011001')  BitMaskRealWorld=Stored Integer
  Out1 : Outport
  wires:
  Bitwise Operator/1 -> Bitwise Operator1/2
  In1/1 -> Bitwise Operator/1
  In2/1 -> Bitwise Operator1/1
  Bitwise Operator1/1 -> Out1/1

== system ES101A_DiagcMgr/DiagcMgr/SetNtcStsCore/NtcNr is Valid/Diagnostics Not Inhibited/NtcEnabled/NTCSTS_PASSD/Update NtcInfoSts /Update NTC Info's Status Byte/CopyRight2 ==

== system ES101A_DiagcMgr/DiagcMgr/SetNtcStsCore/NtcNr is Valid/Diagnostics Not Inhibited/NtcEnabled/NTCSTS_PREFAILD/Update NtcInfoSts, DebCntr and Process RampRate/Deb Counter < MAXDEBCNTRVAL_CNT_S16/Copyright1 ==

== system ES101A_DiagcMgr/DiagcMgr/SetNtcStsCore/NtcNr is Valid/Diagnostics Not Inhibited/NtcEnabled/NTCSTS_PREFAILD/Update NtcInfoSts, DebCntr and Process RampRate/Deb Counter < MAXDEBCNTRVAL_CNT_S16/DebCntr = DebCntr + DebStep ==
  DebStep_ArgIn : Inport
  NtcInfoDebCntr_ArgIn : Inport  Port=2
  Action Port : ActionPort  ActionType=else
  Copyright1 : Subsystem  Description=|  mask(Copyright Information){none=on}
      | Copyright info block.                                               
      |                                                                     
      | Place copyright information at the top of every subsystem in design.
      mask prompts: none "No parameters"
      mask help: Place copyright information at the top of every subsystem in design.
      mask Display:
      | NxtrConf = 'Nexteer Confidential';
      | 
      | sys = bdroot; %handle for the current model ("system")
      | first = get_param(sys,'Created');
      | if(isempty(first))
      |     first = datestr(now,'yyyy');
      | else
      |     first = first(end-3:end);  %year is last four digits
      | end
      | 
      | last = get_param(sys,'LastModifiedDate');
      | if isempty(last)
      |     last = datestr(now,'yyyy');
      | else
      |     last = last(end-3:end);
      | end
      | 
      | if strcmp(first,last)
      |     fprintf('%s\nCopyright  %s Nexteer',NxtrConf,first);
      | else
      |     fprintf('%s\n%s%s-%s Nexteer',NxtrConf,char(169),first,last);
      | end
  Sub : Sum  SaturateOnIntegerOverflow=on
  NtcInfoDebCntr_ArgOut : Outport
  wires:
  Sub/1 -> NtcInfoDebCntr_ArgOut/1
  NtcInfoDebCntr_ArgIn/1 -> Sub/1
  DebStep_ArgIn/1 -> Sub/2

== system ES101A_DiagcMgr/DiagcMgr/SetNtcStsCore/NtcNr is Valid/Diagnostics Not Inhibited/NtcEnabled/NTCSTS_PREFAILD/Update NtcInfoSts, DebCntr and Process RampRate/Deb Counter < MAXDEBCNTRVAL_CNT_S16/DebCntr = DebStep ==
  DebStep_ArgIn : Inport
  Action Port : ActionPort  ActionType=then
  Copyright1 : Subsystem  Description=|  mask(Copyright Information){none=on}
      | Copyright info block.                                               
      |                                                                     
      | Place copyright information at the top of every subsystem in design.
      mask prompts: none "No parameters"
      mask help: Place copyright information at the top of every subsystem in design.
      mask Display:
      | NxtrConf = 'Nexteer Confidential';
      | 
      | sys = bdroot; %handle for the current model ("system")
      | first = get_param(sys,'Created');
      | if(isempty(first))
      |     first = datestr(now,'yyyy');
      | else
      |     first = first(end-3:end);  %year is last four digits
      | end
      | 
      | last = get_param(sys,'LastModifiedDate');
      | if isempty(last)
      |     last = datestr(now,'yyyy');
      | else
      |     last = last(end-3:end);
      | end
      | 
      | if strcmp(first,last)
      |     fprintf('%s\nCopyright  %s Nexteer',NxtrConf,first);
      | else
      |     fprintf('%s\n%s%s-%s Nexteer',NxtrConf,char(169),first,last);
      | end
  NtcInfoDebCntr_ArgOut : Outport
  wires:
  DebStep_ArgIn/1 -> NtcInfoDebCntr_ArgOut/1

== system ES101A_DiagcMgr/DiagcMgr/SetNtcStsCore/NtcNr is Valid/Diagnostics Not Inhibited/NtcEnabled/NTCSTS_PREFAILD/Update NtcInfoSts, DebCntr and Process RampRate/DebCntr = MAXDEBCNTRVAL_CNT_S16/Copyright1 ==

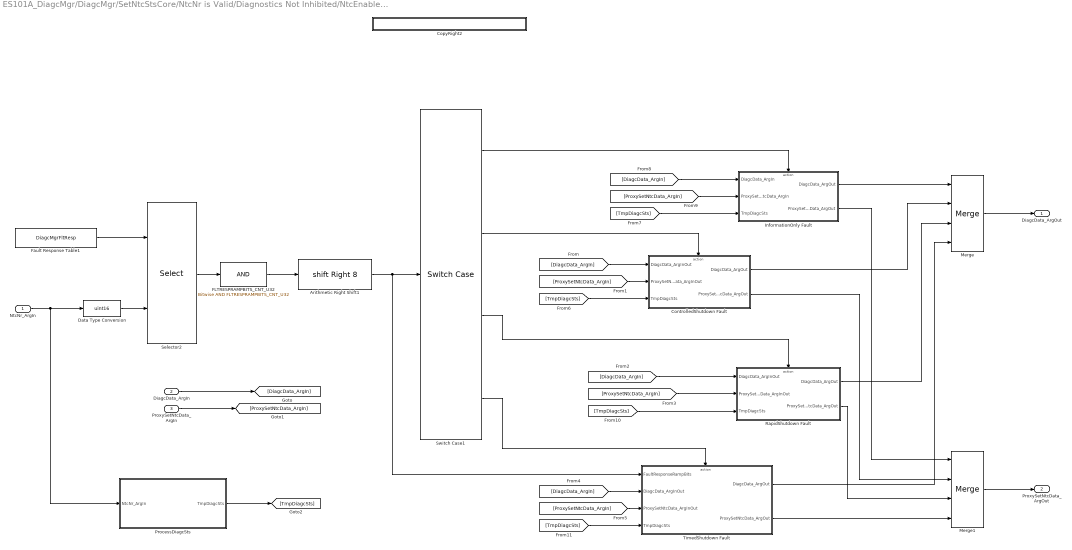
== system ES101A_DiagcMgr/DiagcMgr/SetNtcStsCore/NtcNr is Valid/Diagnostics Not Inhibited/NtcEnabled/NTCSTS_PREFAILD/Update NtcInfoSts, DebCntr and Process RampRate/DebCntr = MAXDEBCNTRVAL_CNT_S16/ProcessRampResponse and DiagcSts ==
  NtcNr_ArgIn : Inport
  DiagcData_ArgIn : Inport  Port=2
  ProxySetNtcData_ArgIn : Inport  Port=3
  Arithmetic Right Shift1 : ArithShift  BitShiftNumber=8  BitShiftDirection=Right
  ControlledShutdown Fault : Subsystem  RequirementInfo={} %GIDa_c2fd7931_695b_44cd_854b_c83a46ea1bdc  TreatAsAtomicUnit=on
  CopyRight2 : Subsystem  Description=|  mask(Copyright Information){none=on}
      | Copyright info block.                                               
      |                                                                     
      | Place copyright information at the top of every subsystem in design.
      mask prompts: none "No parameters"
      mask help: Place copyright information at the top of every subsystem in design.
      mask Display:
      | NxtrConf = 'Nexteer Confidential';
      | 
      | sys = bdroot; %handle for the current model ("system")
      | first = get_param(sys,'Created');
      | first = first(end-3:end);  %year is last four digits
      | 
      | last = get_param(sys,'LastModifiedDate');
      | if isempty(last)
      |     last = datestr(now,'yyyy');
      | else
      |     last = last(end-3:end);
      | end
      | 
      | if strcmp(first,last)
      |     fprintf('%s -- Copyright %s Nexteer',NxtrConf,first)
      | else
      |     fprintf('%s -- %s%s- %s Nexteer',NxtrConf,char(169),first,last)
      | end
  Data Type Conversion : DataTypeConversion  OutDataTypeStr=uint16
  FLTRESPRAMPBITS_CNT_U32 : simulink/Logic and Bit Operations/Bitwise Operator  logicop=AND  UseBitMask=on  BitMask=FLTRESPRAMPBITS_CNT_U32  BitMaskRealWorld=Stored Integer
  Fault Response Table1 : Constant  Value=DiagcMgrFltResp
  InformationOnly Fault : Subsystem  RequirementInfo={} %GIDa_dae963c8_2cc0_4bf3_86a1_a8009b6f9fbb  TreatAsAtomicUnit=on
  Merge : Merge  Inputs=4
  Merge1 : Merge  Inputs=4
  ProcessDiagcSts : Subsystem  RequirementInfo={} %GIDa_86a817ed_81b6_45dd_b9ff_9558a998ec0b
  RapidShutdown Fault : Subsystem  RequirementInfo={} %GIDa_cbdf55f1_97e3_4322_8abb_f07e3ce7d7af  TreatAsAtomicUnit=on
  Selector2 : Selector  IndexMode=Zero-based  InputPortWidth=512  IndexOptions=Index vector (port)  Indices=[1 3]  OutputSizes=1
  Switch Case1 : SwitchCase  CaseConditions={15,14,13}
  TimedShutdown Fault : Subsystem  RequirementInfo={} %GIDa_81505823_09e5_450b_a83b_8437912ec1f5  TreatAsAtomicUnit=on
  DiagcData_ArgOut : Outport
  ProxySetNtcData_ArgOut : Outport  Port=2
  wires:
  NtcNr_ArgIn/1 -> ProcessDiagcSts/1(NtcNr_ArgIn), Data Type Conversion/1
  Arithmetic Right Shift1/1 -> TimedShutdown Fault/1(FaultResponseRampBits), Switch Case1/1
  FLTRESPRAMPBITS_CNT_U32/1 -> Arithmetic Right Shift1/1
  Selector2/1 -> FLTRESPRAMPBITS_CNT_U32/1
  Fault Response Table1/1 -> Selector2/1
  Switch Case1/1 -> InformationOnly Fault/Action
  Switch Case1/2 -> ControlledShutdown Fault/Action
  Switch Case1/3 -> RapidShutdown Fault/Action
  Switch Case1/4 -> TimedShutdown Fault/Action
  Data Type Conversion/1 -> Selector2/2
  DiagcData_ArgIn/1 -> [DiagcData_ArgIn]
  ProxySetNtcData_ArgIn/1 -> [ProxySetNtcData_ArgIn]
  [ProxySetNtcData_ArgIn] -> ControlledShutdown Fault/2(ProxySetNtcData_ArgInOut)
  [DiagcData_ArgIn] -> ControlledShutdown Fault/1(DiagcData_ArgInOut)
  [DiagcData_ArgIn] -> RapidShutdown Fault/1(DiagcData_ArgInOut)
  [ProxySetNtcData_ArgIn] -> RapidShutdown Fault/2(ProxySetNtcData_ArgInOut)
  [DiagcData_ArgIn] -> TimedShutdown Fault/2(DiagcData_ArgInOut)
  [ProxySetNtcData_ArgIn] -> TimedShutdown Fault/3(ProxySetNtcData_ArgInOut)
  Merge/1 -> DiagcData_ArgOut/1
  Merge1/1 -> ProxySetNtcData_ArgOut/1
  ProcessDiagcSts/1(TmpDiagcSts) -> [TmpDiagcSts]
  [TmpDiagcSts] -> InformationOnly Fault/3(TmpDiagcSts)
  [TmpDiagcSts] -> ControlledShutdown Fault/3(TmpDiagcSts)
  [ProxySetNtcData_ArgIn] -> InformationOnly Fault/2(ProxySetNtcData_ArgIn)
  [DiagcData_ArgIn] -> InformationOnly Fault/1(DiagcData_ArgIn)
  [TmpDiagcSts] -> RapidShutdown Fault/3(TmpDiagcSts)
  [TmpDiagcSts] -> TimedShutdown Fault/4(TmpDiagcSts)
  InformationOnly Fault/1(DiagcData_ArgOut) -> Merge/1
  ControlledShutdown Fault/1(DiagcData_ArgOut) -> Merge/2
  RapidShutdown Fault/1(DiagcData_ArgOut) -> Merge/3
  TimedShutdown Fault/1(DiagcData_ArgOut) -> Merge/4
  InformationOnly Fault/2(ProxySetNtcData_ArgOut) -> Merge1/1
  ControlledShutdown Fault/2(ProxySetNtcData_ArgOut) -> Merge1/2
  RapidShutdown Fault/2(ProxySetNtcData_ArgOut) -> Merge1/3
  TimedShutdown Fault/2(ProxySetNtcData_ArgOut) -> Merge1/4

== system ES101A_DiagcMgr/DiagcMgr/SetNtcStsCore/NtcNr is Valid/Diagnostics Not Inhibited/NtcEnabled/NTCSTS_PREFAILD/Update NtcInfoSts, DebCntr and Process RampRate/DebCntr = MAXDEBCNTRVAL_CNT_S16/UpdSnpshtData ==
  NtcNr : Inport
  NtcStInfo : Inport  Port=2
  SnapshotDataBus : Inport  Port=3
  CopyRight1 : Subsystem  Description=|  mask(Copyright Information){none=on}
      | Copyright info block.                                               
      |                                                                     
      | Place copyright information at the top of every subsystem in design.
      mask prompts: none "No parameters"
      mask help: Place copyright information at the top of every subsystem in design.
      mask Display:
      | NxtrConf = 'Nexteer Confidential';
      | 
      | sys = bdroot; %handle for the current model ("system")
      | first = get_param(sys,'Created');
      | first = first(end-3:end);  %year is last four digits
      | 
      | last = get_param(sys,'LastModifiedDate');
      | if isempty(last)
      |     last = datestr(now,'yyyy');
      | else
      |     last = last(end-3:end);
      | end
      | 
      | if strcmp(first,last)
      |     fprintf('%s -- Copyright %s Nexteer',NxtrConf,first)
      | else
      |     fprintf('%s -- %s%s- %s Nexteer',NxtrConf,char(169),first,last)
      | end
  Data Type Conversion : DataTypeConversion  OutDataTypeStr=uint16
  FLTRESPSNPSHTDATAENAD_CNT_U32 : simulink/Logic and Bit Operations/Bitwise Operator  logicop=AND  UseBitMask=on  BitMask=FLTRESPSNPSHTDATAENAD_CNT_U32  BitMaskRealWorld=Stored Integer
  Fault Response Table1 : Constant  Value=DiagcMgrFltResp
  If : If  IfExpression=u1 ~= 0  ShowElse=off
  Selector2 : Selector  IndexMode=Zero-based  InputPortWidth=512  IndexOptions=Index vector (port)  Indices=[1 3]  OutputSizes=1
  Snapshot Data Enabled : Subsystem
  wires:
  NtcNr/1 -> Snapshot Data Enabled/1(NtcNr), Data Type Conversion/1
  Selector2/1 -> FLTRESPSNPSHTDATAENAD_CNT_U32/1
  Fault Response Table1/1 -> Selector2/1
  Data Type Conversion/1 -> Selector2/2
  NtcStInfo/1 -> Snapshot Data Enabled/2(NtcStInfo)
  SnapshotDataBus/1 -> Snapshot Data Enabled/3(SnapshotDataBus)
  FLTRESPSNPSHTDATAENAD_CNT_U32/1 -> If/1
  If/1 -> Snapshot Data Enabled/Action
